simulink model "SourcesExample"  (Simulink 7.5)
settings: Solver=ode45  StartTime=0.0  StopTime=10.0  RelTol=1e-3
libraries: simulink x2
settings Model: Creator=Dranik_win  LastModifiedBy=Dranik_win

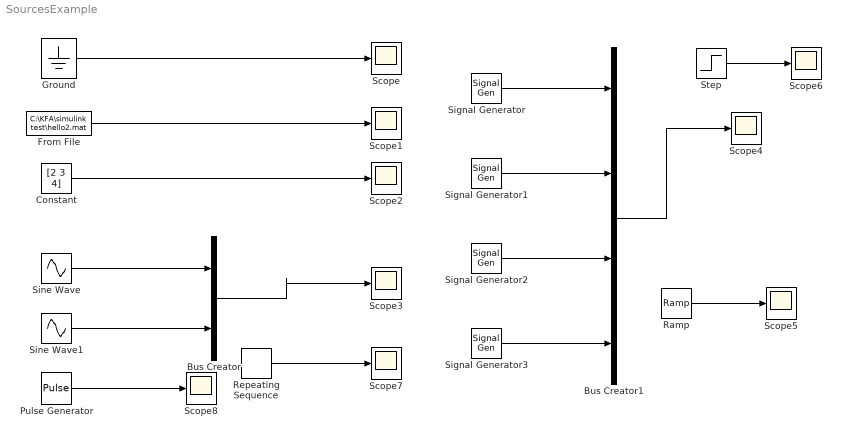
== system SourcesExample ==
  Bus Creator : BusCreator  Inputs=2
  Bus Creator1 : BusCreator
  Constant : Constant  Value=[2 3 4]  OutDataType=fixdt(1, 16)  OutScaling=2^0
  From File : FromFile  FileName=C:\KFA\simulink test\hello2.mat  SampleTime=0
  Ground : Ground
  Pulse Generator : DiscretePulseGenerator  PulseType=Time based  Amplitude=1  Period=10  PulseWidth=5  PhaseDelay=4  SampleTime=1
  Ramp : simulink/Sources/Ramp  SystemSampleTime=-1  slope=0.05  start=2  X0=2
  Repeating Sequence : simulink/Sources/Repeating Sequence  SystemSampleTime=-1  rep_seq_t=[0 1 2]  rep_seq_y=[0 2 2]
  Scope{,1..8} (9 alike) : Scope
      Scope2 settings: SaveName=ScopeData2
      Scope3 settings: SaveName=ScopeData3
      Scope4 settings: SaveName=ScopeData4
      Scope5 settings: SaveName=ScopeData5
      Scope6 settings: SaveName=ScopeData6
      Scope7 settings: SaveName=ScopeData7
      Scope8 settings: SaveName=ScopeData8
  Signal Generator : SignalGenerator
  Signal Generator1 : SignalGenerator  WaveForm=square  Amplitude=3
  Signal Generator2 : SignalGenerator  WaveForm=sawtooth
  Signal Generator3 : SignalGenerator  WaveForm=random
  Sine Wave : Sin  Amplitude=0.5  Bias=0  Frequency=1  Phase=0  Samples=10  SampleTime=0  Offset=0
  Sine Wave1 : Sin  Amplitude=2  Bias=1  Frequency=3  Phase=1  Samples=10  SampleTime=0  Offset=0
  Step : Step  Time=3  SampleTime=3
  wires:
  Ground/1 -> Scope/1
  From File/1 -> Scope1/1
  Constant/1 -> Scope2/1
  Bus Creator/1 -> Scope3/1
  Sine Wave/1 -> Bus Creator/1
  Sine Wave1/1 -> Bus Creator/2
  Signal Generator/1 -> Bus Creator1/1
  Bus Creator1/1 -> Scope4/1
  Signal Generator1/1 -> Bus Creator1/2
  Signal Generator2/1 -> Bus Creator1/3
  Signal Generator3/1 -> Bus Creator1/4
  Ramp/1 -> Scope5/1
  Step/1 -> Scope6/1
  Repeating Sequence/1 -> Scope7/1
  Pulse Generator/1 -> Scope8/1
